simulink model "sampleModel10"  (R2021b)
settings: Solver=VariableStepAuto  StartTime=0.0  StopTime=10.0  RelTol=1e-3
undefined symbols (not defined in the file or in its folder): DiscIntNeverNeededParam, Newton, Raphson
libraries: simulink x4
settings Model: Creator=user  LastModifiedBy=user

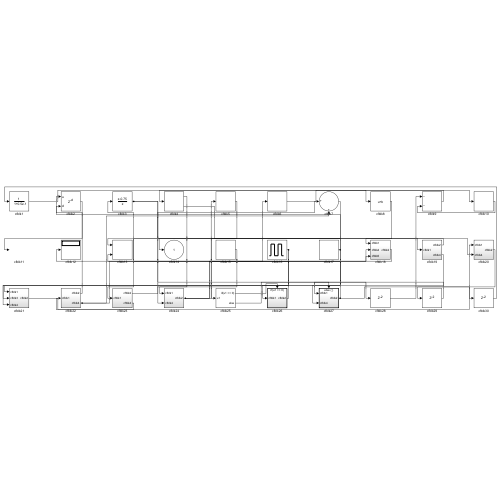
[thumbnail: Simulink's stored preview of the top-level diagram]
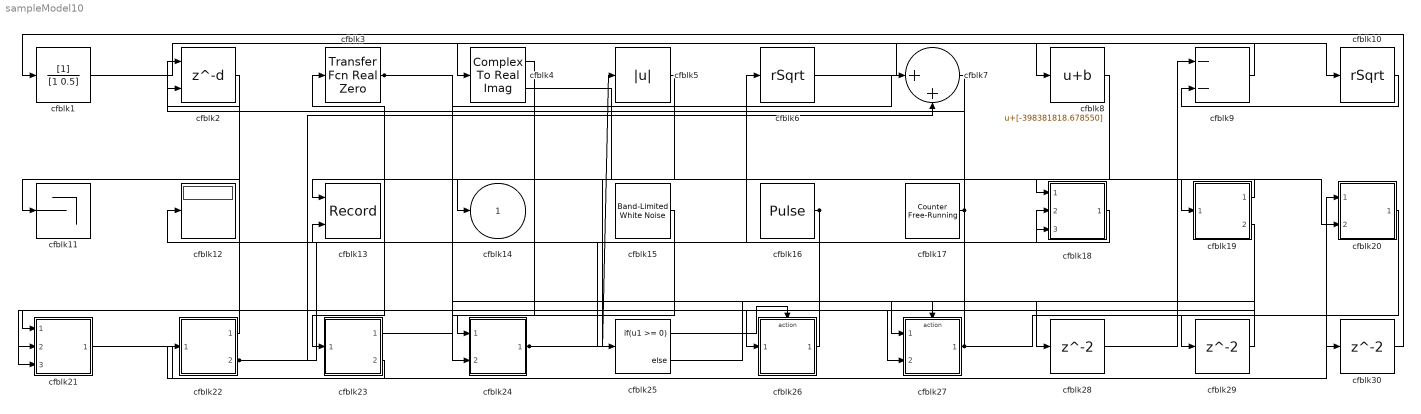
== system sampleModel10 ==
  cfblk1 : DiscreteFilter  SampleTime=1
  cfblk10 : Sqrt  Operator=rSqrt  AlgorithmType=Newton-Raphson  SaturateOnIntegerOverflow=on
  cfblk11 : Terminator
  cfblk12 : Display
  cfblk13 : Record  FileSettingsInternal="{\"entries\":[{\"content\":{\"excelSettings\":{\"content\":{},\"type\":\"Streamout.ExcelSettings\"}},\"type\":\"Streamout.FileSettingStorage\",\"uuid\":\"12464234-0123-4500-b757-1bcb142e4388\"}],\"packageUris\":[\"http://schema.mathworks.com/mf0/streamout_blocks/R2020a\"],\"version\":\"1.0\"}"  Layout=[1 1]  SignalsInternal="{\"entries\":[{\"content\":{\"signals\":[{\"content\":{\"blockPath\":[\"sampleModel10/cfblk13\"],\"channel\":[],\"dimensions\":[1],\"domain\":\"sampleModel10/cfblk13\",\"lineColor\":\"#a2142f\",\"plots\":[1],\"port\":1,\"sid\":[\"\"],\"signalID\":351,\"signalName\":\"cfblk7\"},\"type\":\"RecordBlkView.Signal\",\"uuid\":\"addf4039-dc77-4d44-b335-c1f742a5f9f0\"},{\"content\":{\"blockPath\":[\"sampleModel10/cfblk13\"],\"channel\":[],\"dimensions\":[1],\"domain\":\"sampleModel10/cfblk13\",\"lineColor\":\"#139fff\",\"plots\":[1],\"port\":2,\"sid\":[\"\"],\"signalID\":355,\"signalName\":\"cfblk18\"},\"type\":\"RecordBlkView.Signal\",\"uuid\":\"525077b9-96c4-4f52-bbb1-824d5e901206\"}]},\"type\":\"RecordBlkView.InputSignals\",\"uuid\":\"c7a7e27a-2a1e-411f-b053-04083caf397b\"}],\"packageUris\":[\"http://schema.mathworks.com/mf0/streamout_blocks/R2020a\"],\"version\":\"1.0\"}"  VisualizationBindings="{\"xyplotplugin\":{\"info\":[{\"series\":[{\"bindingParametersList\":[{\"parameter\":\"X-Axis\",\"signalID\":351,\"signalName\":\"cfblk7\"},{\"parameter\":\"Y-Axis\",\"signalID\":355,\"signalName\":\"cfblk18\"}],\"seriesID\":13934}],\"subplotID\":1}]}}"  CompatibilityTag=XY
  cfblk15 : simulink/Sources/Band-Limited White Noise  Cov=[3510984324.794902]  Ts=0.1  seed=[542973539.000000]
  cfblk16 : DiscretePulseGenerator  PulseType=Time based  Amplitude=[417409233.958450]  Period=[99292844.137471]  PulseWidth=5  PhaseDelay=[2.000000]
  cfblk17 : simulink/Sources/Counter Free-Running  NumBits=[7.000000]  tsamp=-1
  cfblk18 : Subsystem
  cfblk19 : Subsystem
  cfblk2 : Delay  DelayLengthSource=Input port  SampleTime=1
      settings: InputPortMap=u0,p1
  cfblk20 : Subsystem
  cfblk21 : Subsystem
  cfblk22 : Subsystem
  cfblk23 : Subsystem
  cfblk24 : Subsystem
  cfblk25 : If  IfExpression=u1 >= 0  SampleTime=1
  cfblk26 : Subsystem  TreatAsAtomicUnit=on
  cfblk27 : Subsystem  TreatAsAtomicUnit=on
  cfblk28 : Delay  SampleTime=1
  cfblk29 : Delay  SampleTime=1
  cfblk3 : simulink/Discrete/Transfer Fcn Real Zero  ZeroZ=0.75  ICPrevInput=0.0  DoSatur=off
      settings: SourceProductBaseCode=SL
  cfblk30 : Delay  SampleTime=1
  cfblk4 : ComplexToRealImag
  cfblk5 : Abs
  cfblk6 : Sqrt  Operator=rSqrt  AlgorithmType=Newton-Raphson  SaturateOnIntegerOverflow=on
  cfblk7 : Sum  Inputs=|++
  cfblk8 : Bias  Bias=[-398381818.678550]
  cfblk9 : Sum  Inputs=--
  cfblk14 : Outport
  wires:
  cfblk7/1 -> cfblk13/1
  cfblk18/1(cfblk2) -> cfblk13/2
  cfblk1/1 -> cfblk10/1
  cfblk16/1 -> cfblk21/1(cfblk1), cfblk26/1(cfblk1)
  cfblk3/1 -> cfblk20/2(cfblk4), cfblk28/1
  cfblk6/1 -> cfblk8/1
  cfblk24/1(cfblk2) -> cfblk5/1, cfblk18/2(cfblk4), cfblk18/3(cfblk5)
  cfblk2/1 -> cfblk11/1
  cfblk22/1(cfblk2) -> cfblk12/1
  cfblk26/1(cfblk2) -> cfblk3/1
  cfblk10/1 -> cfblk9/2
  cfblk22/2(cfblk4) -> cfblk6/1, cfblk7/2
  cfblk27/1(cfblk2) -> cfblk2/1, cfblk30/1
  cfblk9/1 -> cfblk4/1
  cfblk5/1 -> cfblk23/1(cfblk1)
  cfblk21/1(cfblk2) -> cfblk20/1(cfblk1)
  cfblk15/1 -> cfblk24/1(cfblk1)
  cfblk17/1 -> cfblk14/1, cfblk2/2, cfblk21/2(cfblk3), cfblk21/3(cfblk4)
  cfblk23/1(cfblk2) -> cfblk7/1
  cfblk23/2(cfblk4) -> cfblk22/1(cfblk1)
  cfblk8/1 -> cfblk25/1
  cfblk19/1(cfblk2) -> cfblk18/1(cfblk1)
  cfblk19/2(cfblk4) -> cfblk27/2(cfblk4)
  cfblk4/1 -> cfblk24/2(cfblk4)
  cfblk4/2 -> cfblk19/1(cfblk1)
  cfblk25/1 -> cfblk26/Action
  cfblk25/2 -> cfblk27/Action
  cfblk28/1 -> cfblk9/1
  cfblk20/1(cfblk2) -> cfblk29/1
  cfblk29/1 -> cfblk27/1(cfblk1)
  cfblk30/1 -> cfblk1/1

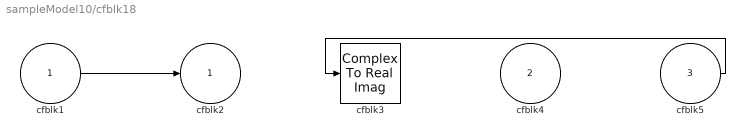
== system sampleModel10/cfblk18 ==
  cfblk1 : Inport
  cfblk4 : Inport  Port=2
  cfblk5 : Inport  Port=3
  cfblk3 : ComplexToRealImag
  cfblk2 : Outport
  wires:
  cfblk1/1 -> cfblk2/1
  cfblk5/1 -> cfblk3/1

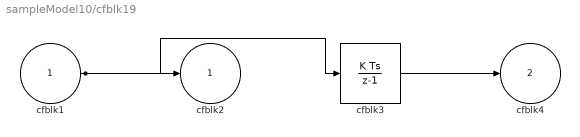
== system sampleModel10/cfblk19 ==
  cfblk1 : Inport
  cfblk3 : DiscreteIntegrator  ICPrevOutput=DiscIntNeverNeededParam  ICPrevScaledInput=DiscIntNeverNeededParam
  cfblk2 : Outport
  cfblk4 : Outport  Port=2
  wires:
  cfblk1/1 -> cfblk2/1, cfblk3/1
  cfblk3/1 -> cfblk4/1

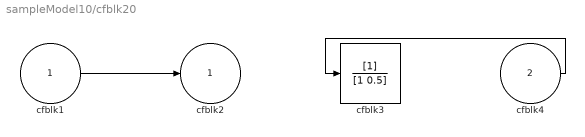
== system sampleModel10/cfblk20 ==
  cfblk1 : Inport
  cfblk4 : Inport  Port=2
  cfblk3 : DiscreteFilter  SampleTime=1
  cfblk2 : Outport
  wires:
  cfblk1/1 -> cfblk2/1
  cfblk4/1 -> cfblk3/1

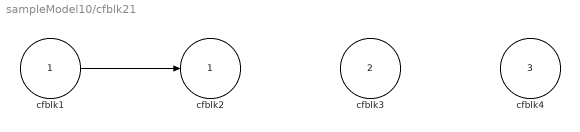
== system sampleModel10/cfblk21 ==
  cfblk1 : Inport
  cfblk3 : Inport  Port=2
  cfblk4 : Inport  Port=3
  cfblk2 : Outport
  wires:
  cfblk1/1 -> cfblk2/1

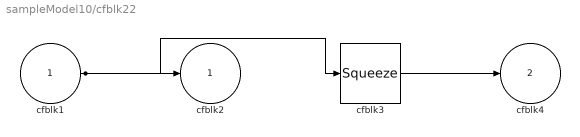
== system sampleModel10/cfblk22 ==
  cfblk1 : Inport
  cfblk3 : Squeeze
  cfblk2 : Outport
  cfblk4 : Outport  Port=2
  wires:
  cfblk3/1 -> cfblk4/1
  cfblk1/1 -> cfblk2/1, cfblk3/1

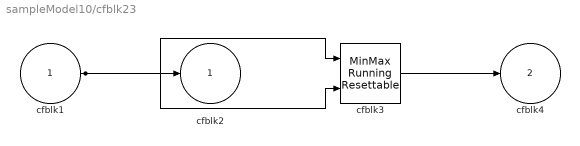
== system sampleModel10/cfblk23 ==
  cfblk1 : Inport
  cfblk3 : simulink/Math Operations/MinMax Running Resettable  Function=min  vinit=0.0
  cfblk2 : Outport
  cfblk4 : Outport  Port=2
  wires:
  cfblk3/1 -> cfblk4/1
  cfblk1/1 -> cfblk2/1, cfblk3/1, cfblk3/2

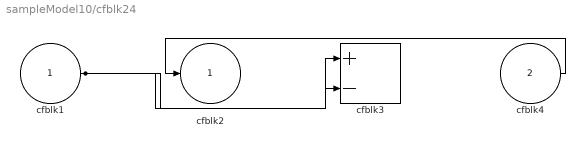
== system sampleModel10/cfblk24 ==
  cfblk1 : Inport
  cfblk4 : Inport  Port=2
  cfblk3 : Sum  Inputs=+-
  cfblk2 : Outport
  wires:
  cfblk4/1 -> cfblk2/1
  cfblk1/1 -> cfblk3/1, cfblk3/2

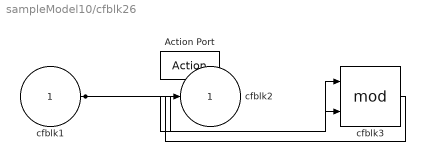
== system sampleModel10/cfblk26 ==
  cfblk1 : Inport
  Action Port : ActionPort  ActionPortLabel=if(u1 >= 0)
  cfblk3 : Math  Operator=mod  SaturateOnIntegerOverflow=on
  cfblk2 : Outport
  wires:
  cfblk1/1 -> cfblk3/1, cfblk3/2
  cfblk3/1 -> cfblk2/1

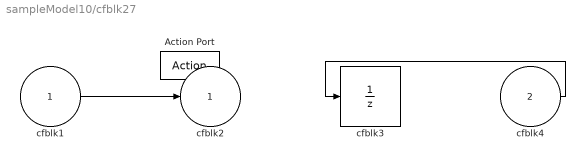
== system sampleModel10/cfblk27 ==
  cfblk1 : Inport
  cfblk4 : Inport  Port=2
  Action Port : ActionPort  ActionPortLabel=else
  cfblk3 : UnitDelay  SampleTime=-1  HasFrameUpgradeWarning=on
  cfblk2 : Outport
  wires:
  cfblk1/1 -> cfblk2/1
  cfblk4/1 -> cfblk3/1
